simulink model "APP_Kickdown"  (R2016b)
settings: configuration reference "CodeGenConfigSet" (kept outside this file)
values from neighbouring files (symbols this model uses):
  APP_uKDHighAPP_C = Calibration.Parameter    [init_APP_Kickdown.m]
  APP_uKDLowAPP_C = Calibration.Parameter    [init_APP_Kickdown.m]
  MoFAPP_dRawSigFac_C = Calibration.Parameter    [init_APP_Kickdown.m]
  SigTst_stAPPKickDown_C = Calibration.Parameter    [init_APP_Kickdown.m]
  SigTst_swtAPPKickDown_C = Calibration.Parameter    [init_APP_Kickdown.m]
undefined symbols (not defined in the file or in its folder): Switch_conv
libraries: CXLib x2
settings Model: Creator=lenovo  LastModifiedBy=lenovo
settings ConfigSetRef: SourceLocation=Base Workspace

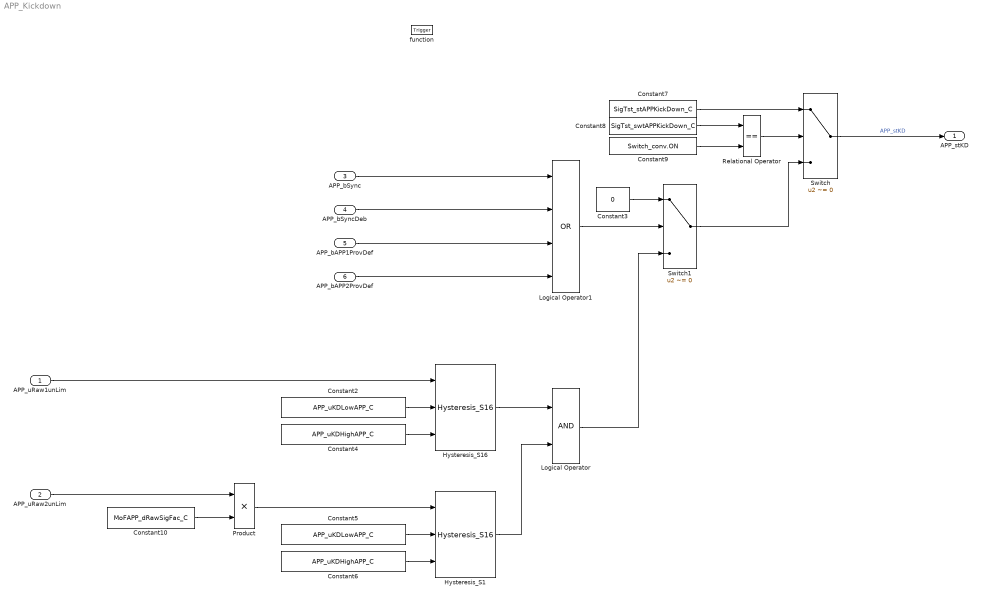
== system APP_Kickdown ==
  APP_uRaw1unLim : Inport  Tag=mv  Description=Acceleration pedal sensor 1 unlimited raw value  OutMin=0  OutMax=5000  OutDataTypeStr=Ad_mv
  APP_uRaw2unLim : Inport  Tag=mv  Description=Acceleration pedal sensor 2 unlimited raw value  Port=2  OutMin=0  OutMax=5000  OutDataTypeStr=Ad_mv
  APP_bSync : Inport  Description=Status temporary sync check  Port=3  OutMin=0  OutMax=1  OutDataTypeStr=boolean
  APP_bSyncDeb : Inport  Description=Status debounced sync check  Port=4  OutMin=0  OutMax=1  OutDataTypeStr=boolean
  APP_bAPP1ProvDef : Inport  Description=Status Sensor 1 of the acceleration pedal temporary defect  Port=5  OutMin=0  OutMax=1  OutDataTypeStr=boolean
  APP_bAPP2ProvDef : Inport  Description=Status Sensor 2 of the acceleration pedal temporary defect  Port=6  OutMin=0  OutMax=1  OutDataTypeStr=boolean
  function : TriggerPort  TriggerType=function-call  VariantControl=Variant
  Constant10 : Constant  Value=MoFAPP_dRawSigFac_C  SampleTime=-1
  Constant2 : Constant  RequirementInfo={'other' 'APP_requirements.doc' '@Simulink_requirement_item_11' 'true' '识别策略。' '' } %GIDa_de88adba_cd32_4ac1_86f6_6a9e99d467a8  Value=APP_uKDLowAPP_C
  Constant3 : Constant  Value=0  OutDataTypeStr=Inherit: Inherit via back propagation
  Constant4 : Constant  RequirementInfo={'other' 'APP_requirements.doc' '@Simulink_requirement_item_11' 'true' '识别策略。' '' } %GIDa_47907319_ec30_4af5_b4e0_03ab52ea1e63  Value=APP_uKDHighAPP_C
  Constant5 : Constant  RequirementInfo={'other' 'APP_requirements.doc' '@Simulink_requirement_item_11' 'true' '识别策略。' '' } %GIDa_0b6facfb_ed1b_40e2_aef7_84b1aec06b0d  Value=APP_uKDLowAPP_C
  Constant6 : Constant  RequirementInfo={'other' 'APP_requirements.doc' '@Simulink_requirement_item_11' 'true' '识别策略。' '' } %GIDa_963c08aa_135d_41fb_aedc_0f8bc8a7126a  Value=APP_uKDHighAPP_C
  Constant7 : Constant  RequirementInfo={'other' 'APP_requirements.doc' '@Simulink_requirement_item_12' 'true' '手动开关。' '' } %GIDa_746c51a7_309d_463b_9d12_5b1bf86154e9  Value=SigTst_stAPPKickDown_C
  Constant8 : Constant  RequirementInfo={'other' 'APP_requirements.doc' '@Simulink_requirement_item_12' 'true' '手动开关。' '' } %GIDa_2b07b4bb_f1ee_4bd0_9203_6758ef3ff403  Value=SigTst_swtAPPKickDown_C
  Constant9 : Constant  RequirementInfo={'other' 'APP_requirements.doc' '@Simulink_requirement_item_12' 'true' '手动开关。' '' } %GIDa_f490a52b_783e_493c_befd_fa6d0ab33dc7  Value=Switch_conv.ON  OutDataTypeStr=Inherit: Inherit via back propagation
  Hysteresis_S1 : CXLib/Hysteresis_S16  RequirementInfo={'other' 'APP_requirements.doc' '@Simulink_requirement_item_11' 'true' '识别策略。' '' } %GIDa_62f1f87e_92e6_4181_801e_4b26282d5168
  Hysteresis_S16 : CXLib/Hysteresis_S16  RequirementInfo={'other' 'APP_requirements.doc' '@Simulink_requirement_item_11' 'true' '识别策略。' '' } %GIDa_6b887cd7_f6f3_4fb8_9dc7_374f677a1c0f
  Logical Operator : Logic  RequirementInfo={'other' 'APP_requirements.doc' '@Simulink_requirement_item_11' 'true' '识别策略。' '' } %GIDa_cc37cddb_5ff6_4886_beef_2e304e3068fe  OutDataTypeStr=boolean
  Logical Operator1 : Logic  Operator=OR  Inputs=4  OutDataTypeStr=boolean
  Product : Product  RequirementInfo={'other' 'APP_requirements.doc' '@Simulink_requirement_item_11' 'true' '识别策略。' '' } %GIDa_81017875_13a2_440d_9998_03a589d9e080  OutDataTypeStr=Ad_mv
  Relational Operator : RelationalOperator  Operator===  OutDataTypeStr=boolean  RndMeth=Simplest
  Switch : Switch  RequirementInfo={'other' 'APP_requirements.doc' '@Simulink_requirement_item_12' 'true' '手动开关。' '' } %GIDa_2033430e_1174_4155_b1e8_dd3f3154609c  Criteria=u2 ~= 0  InputSameDT=on
  Switch1 : Switch  Criteria=u2 ~= 0  InputSameDT=on
  APP_stKD : Outport  Description=State of accelerator pedal kick down  OutMin=0  OutMax=1  OutDataTypeStr=boolean
  wires:
  Constant10/1 -> Product/2
  Constant9/1 -> Relational Operator/2
  APP_bAPP2ProvDef/1 -> Logical Operator1/4
  APP_bAPP1ProvDef/1 -> Logical Operator1/3
  APP_bSyncDeb/1 -> Logical Operator1/2
  APP_bSync/1 -> Logical Operator1/1
  APP_uRaw2unLim/1 -> Product/1
  Switch1/1 -> Switch/3
  Logical Operator/1 -> Switch1/3
  Relational Operator/1 -> Switch/2
  Constant7/1 -> Switch/1
  Constant8/1 -> Relational Operator/1
  Product/1 -> Hysteresis_S1/1
  Hysteresis_S16/1 -> Logical Operator/1
  Hysteresis_S1/1 -> Logical Operator/2
  Constant6/1 -> Hysteresis_S1/3
  Constant5/1 -> Hysteresis_S1/2
  Constant2/1 -> Hysteresis_S16/2
  Constant4/1 -> Hysteresis_S16/3
  APP_uRaw1unLim/1 -> Hysteresis_S16/1
  Constant3/1 -> Switch1/1
  Logical Operator1/1 -> Switch1/2
  Switch/1 -> APP_stKD/1  "APP_stKD"
